simulink model "nav_filter"  (R2025b)
settings: Solver=ode4  StartTime=0.0  StopTime=50  FixedStep=ST  RelTol=1e-3
InitFcn:
  | addpath(genpath('KF_utilities'));
values from neighbouring files (symbols this model uses):
  acc = acc_f    [TRAJECTORY1.m]
  bias_gyro = [1 1 1]    [TRAJECTORY1.m]
  g = Simulink.Parameter    [TRAJECTORY1.m]
  P_bases_ned = Simulink.Parameter    [TRAJECTORY1.m]
  pos = pos_f    [TRAJECTORY1.m]
  pqr = omega_n    [TRAJECTORY1.m]
  Q = Simulink.Parameter    [TRAJECTORY1.m]
  quat_nb = compact(quat)    [TRAJECTORY1.m]
  sensor_covariances = Simulink.Parameter    [TRAJECTORY1.m]
  ST = 1/100    (= 0.01)    [TRAJECTORY1.m]    (also in WP_High_acc.m; WP_low_acc.m)
  vel_ned = vel_n_f    [TRAJECTORY1.m]
undefined symbols (not defined in the file or in its folder): DiscIntNeverNeededParam, freq_gyro, freq_UWB, N_bases, std_dev_gyro1, std_dev_gyro2, std_dev_gyro3, std_dev_magx, std_dev_magy, std_dev_magz, std_dev_UWB1, Tf
libraries: cstblocks x8, simulink x1
settings Model: Creator=eugde  LastModifiedBy=eugde

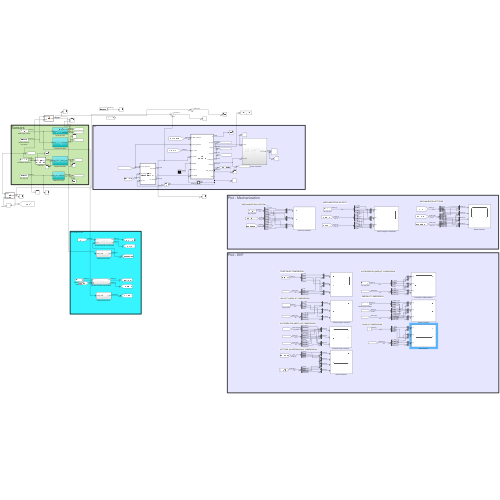
[thumbnail: Simulink's stored preview of the top-level diagram]
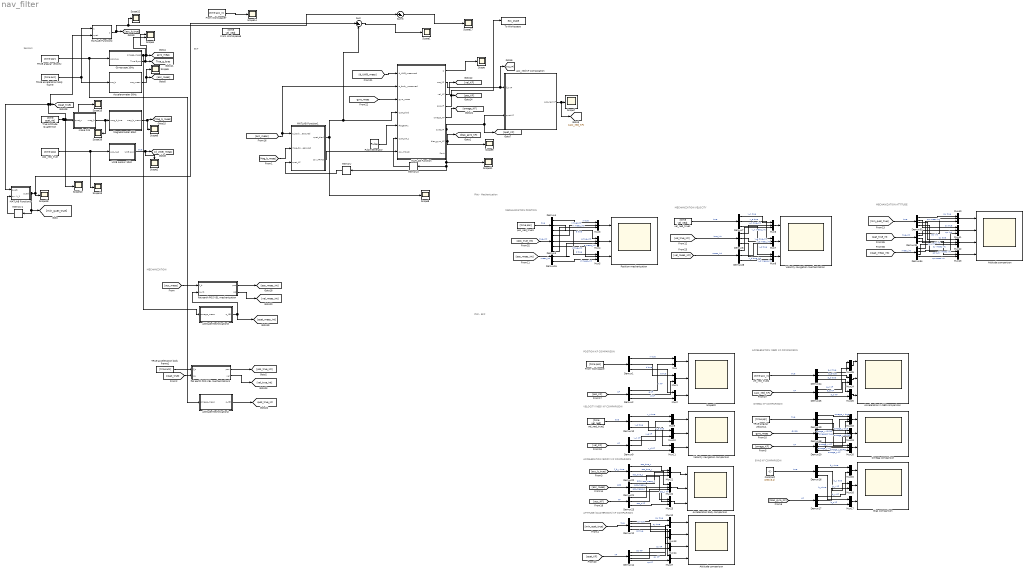
== system nav_filter ==
  note: MECHANIZATION
  note: EKF
  note: Sensors
  note: VELOCITY (NED) KF COMPARISON
  note: Plot - Mechanization
  note: MECHANIZATION VELOCITY
  note: OMEGA KF COMPARISON
  note: ACCELERATION (BODY) KF COMPARISON
  note: Plot - EKF
  note: POSITION KF COMPARISON
  note: MECHANIZATION POSITION
  note: BYAS KF COMPARISON
  note: ACCELERATION (NED) KF COMPARISON
  note: MECHANIZATION ATTITUDE
  note: ATTITUDE (QUATERNION) KF COMPARISON
  Acceleration body comparison : Scope  NumInputPorts=3
      settings: ActiveDisplayYMinimum=-4.52669  ActiveDisplayYMaximum=3.39128  YLabel=acc_x [m/s^2]
  Acceleration in NED comparison : Scope  NumInputPorts=3
      settings: ActiveDisplayYMinimum=-1.28826  ActiveDisplayYMaximum=1.68364  YLabel=acc_n [m/s^2]  DataLoggingVariableName=ScopeData2
  Accelerometer 50Hz : Subsystem
  Attitude Mechnization2 : Subsystem
  Attitude Mechnization3 : Subsystem
  "Attitude comparison " : Scope  NumInputPorts=4
      settings: ActiveDisplayYMinimum=-0.55605  ActiveDisplayYMaximum=1.17289  YLabel=qw  DataLoggingVariableName=ScopeData4
  "Attitude comparison " : Scope  NumInputPorts=4
      settings: ActiveDisplayYMinimum=-0.59703  ActiveDisplayYMaximum=1.17766  YLabel=qw  DataLoggingVariableName=ScopeData5
  Bias comparison : Scope  NumInputPorts=3
      settings: ActiveDisplayYMinimum=0.42457  ActiveDisplayYMaximum=1.1239  YLabel=bias_x [rad/s]  DataLoggingVariableName=ScopeData6
  Constant : Constant  Value=ones(3,1)
  Demux{1..4,6..7,9..10,15..25,28} (20 alike) : Demux  Outputs=3
  Demux{12,14,32..34} (5 alike) : Demux
  From Workspace : FromWorkspace  VariableName=[time pos]
  From Workspace6 : FromWorkspace  VariableName=[time vel_ned]
  From Workspace7 : FromWorkspace  VariableName=[time acc_n]
  Gyroscope 10Hz : Subsystem
  MATLAB Function : MATLAB Function  InitFcn=addpath('C:\Users\eugde\OneDrive\Documenti\Uni Pisa\Esami\SGN\PROGETTO\KF_utilities')  TreatAsAtomicUnit=on
  MATLAB Function1 : MATLAB Function  TreatAsAtomicUnit=on
  MATLAB Function2 : MATLAB Function  TreatAsAtomicUnit=on
  MATLAB Function3 : MATLAB Function  TreatAsAtomicUnit=on
  Magnetometer 50Hz : Subsystem
  Memory : Memory
  Memory1 : Memory  InitialCondition=quat_nb(1,:)
  Memory2 : Memory  InitialCondition=[1 0 0 0]'
  Mux{,1..2,9..17,24..27} (16 alike) : Mux  Inputs=2
  Mux{3..8,18..23,40..43} (16 alike) : Mux  Inputs=3
  Omega comparison : Scope  NumInputPorts=3
      settings: ActiveDisplayYMinimum=-0.27702  ActiveDisplayYMaximum=1.31187  YLabel=omega_x [rad/s]  DataLoggingVariableName=ScopeData7
  Position mechanization : Scope  NumInputPorts=3
      settings: ActiveDisplayYMinimum=-9.13016  ActiveDisplayYMaximum=45.84035  YLabel=North [m]  DataLoggingVariableName=ScopeData8
  Pulse Generator : DiscretePulseGenerator  PulseType=Time based  Period=1/50  PulseWidth=50
  Scope{,1..2,5..18} (17 alike) : Scope
      Scope settings: ActiveDisplayYMinimum=726.13831  ActiveDisplayYMaximum=1136.65509
      Scope1 settings: ActiveDisplayYMinimum=-0.05537  ActiveDisplayYMaximum=0.0472
      Scope10 settings: ActiveDisplayYMinimum=-1.54993  ActiveDisplayYMaximum=1.58064
      Scope11 settings: ActiveDisplayYMinimum=-0.44551  ActiveDisplayYMaximum=1.21227  DataLoggingVariableName=ScopeData12
      Scope12 settings: ActiveDisplayYMinimum=-0.13409  ActiveDisplayYMaximum=0.09726  DataLoggingVariableName=ScopeData13
      Scope13 settings: ActiveDisplayYMinimum=-15.92056  ActiveDisplayYMaximum=36.67619  DataLoggingVariableName=ScopeData14
      Scope14 settings: ActiveDisplayYMinimum=-4.68451  ActiveDisplayYMaximum=4.54841  DataLoggingVariableName=ScopeData2
      Scope15 settings: ActiveDisplayYMinimum=-0.55552  ActiveDisplayYMaximum=1.17284
      Scope16 settings: ActiveDisplayYMinimum=-0.9809  ActiveDisplayYMaximum=1.11497  DataLoggingVariableName=ScopeData2
      Scope17 settings: ActiveDisplayYMinimum=-9.00868  ActiveDisplayYMaximum=9.03518  DataLoggingVariableName=ScopeData2
      Scope18 settings: ActiveDisplayYMinimum=-0.55552  ActiveDisplayYMaximum=1.17284
      Scope2 settings: ActiveDisplayYMinimum=1.85826  ActiveDisplayYMaximum=83.14894  DataLoggingVariableName=ScopeData4
      Scope5 settings: ActiveDisplayYMinimum=-11.04684  ActiveDisplayYMaximum=1.25671  DataLoggingVariableName=ScopeData6
      Scope6 settings: ActiveDisplayYMinimum=-0.9809  ActiveDisplayYMaximum=1.11497  DataLoggingVariableName=ScopeData7
      Scope7 settings: ActiveDisplayYMinimum=-0.90235  ActiveDisplayYMaximum=0.76851  DataLoggingVariableName=ScopeData3
      Scope8 settings: ActiveDisplayYMinimum=-1.24871  ActiveDisplayYMaximum=1.24986
      Scope9 settings: ActiveDisplayYMinimum=0.05252  ActiveDisplayYMaximum=2.64364  DataLoggingVariableName=ScopeData5
  Scope20 : Scope  NumInputPorts=3
      settings: ActiveDisplayYMinimum=-3.73177  ActiveDisplayYMaximum=33.62683  YLabel=North  DataLoggingVariableName=ScopeData9
  Scope4 : Scope  NumInputPorts=2
      settings: ActiveDisplayYMinimum=0.99965  ActiveDisplayYMaximum=1.00021  DataLoggingVariableName=ScopeData5
  Sum : Sum  Inputs=|+-
  Sum3 : Sum  Inputs=|+-
  TRUE acceleration body frame : FromWorkspace  VariableName=[time acc]  SampleTime=ST
  TRUE acceleration body frame1 : FromWorkspace  VariableName=[time acc]  SampleTime=ST
  TRUE angular velocity : FromWorkspace  VariableName=[time pqr]  SampleTime=ST
  TRUE angular velocity1 : FromWorkspace  VariableName=[time pqr]  SampleTime=ST
  To Workspace : ToWorkspace  VariableName=ecs_state  SaveFormat=Structure With Time  SampleTime=-1
  True Attitude Quaternion : FromWorkspace  VariableName=[time quat_nb]  SampleTime=ST
  UWB sensor 10Hz : Subsystem
  Velocity navigation comparison : Scope  NumInputPorts=3
      settings: ActiveDisplayYMinimum=-0.23511  ActiveDisplayYMaximum=1.32366  YLabel=vel_n [m/s]  DataLoggingVariableName=ScopeData10
  Velocity navigation mechanization : Scope  NumInputPorts=3
      settings: ActiveDisplayYMinimum=0.32185  ActiveDisplayYMaximum=0.95452  YLabel=vel_n [m/s]  DataLoggingVariableName=ScopeData11
  "acc_ned KF computation " : Subsystem
  flat earth POS VEL mechanization : Subsystem
  flat earth POS VEL mechanization1 : Subsystem
  make Cnb : MATLAB Function  TreatAsAtomicUnit=on
  pos_ned_true : FromWorkspace  VariableName=[time pos]  SampleTime=ST
  pos_ned_true1 : FromWorkspace  VariableName=[time pos]  SampleTime=ST
  vel_ned_true1 : FromWorkspace  VariableName=[time vel_ned]  SampleTime=ST
  vel_ned_true2 : FromWorkspace  VariableName=[time vel_ned]  SampleTime=ST
  vel_ned_true4 : FromWorkspace  VariableName=[time acc_n]  SampleTime=ST
  tag scope: True_g_byas=global, gyro_meas=global, quat_true_int=global
  wires:
  Magnetometer 50Hz/1(mag_b_meas) -> Scope6/1, [Mag_b_meas]
  True Attitude Quaternion/1 -> Scope10/1, MATLAB Function3/1("quatk "), MATLAB Function2/2(quat), [quat_true], Scope15/1, make Cnb/1(quat_n)
  Gyroscope 10Hz/2(True Byas) -> Scope4/2, [True_g_byas]
  Gyroscope 10Hz/1(omega_meas) -> Attitude Mechnization3/1(omega_meas), [gyro_meas], Scope4/1
  pos_ned_true/1 -> Scope13/1, UWB sensor 10Hz/1(pos_ned)
  Accelerometer 50Hz/1(acc_meas) -> Scope5/1, [acc_meas]
  TRUE angular velocity/1 -> Attitude Mechnization2/1(omega_meas), Gyroscope 10Hz/1(pqr_true)
  TRUE acceleration body frame/1 -> MATLAB Function2/1(acc_meas), Accelerometer 50Hz/1(acc_b)
  UWB sensor 10Hz/1("UWB pos ") -> Scope2/1, [d_UWB_meas]  "true"
  "acc_ned KF computation "/1(acc_ned KF) -> [acc_ned_KF], Scope7/1
  MATLAB Function/6(quat_KF) -> Scope11/1, Memory2/1, Memory/1, [quat_KF], "acc_ned KF computation "/2(quat KF)
  [acc_meas] -> MATLAB Function/2(a_body_measured), MATLAB Function1/1(a_body_measured)
  MATLAB Function/7(bias_gyro_KF) -> [bias_gyro_KF], Scope9/1
  MATLAB Function/5(omega_KF) -> [omega_KF]
  MATLAB Function/4(pos_KF) -> To Workspace/1, [pos_KF]
  [gyro_meas] -> MATLAB Function/3(gyro_meas)
  [d_UWB_meas] -> MATLAB Function/1(d_UWB_measured)
  make Cnb/1(mag_b) -> Scope16/1, Magnetometer 50Hz/1(mag_b_true)
  MATLAB Function1/1(quat_triad) -> Scope8/1, Sum/2, MATLAB Function/4(quat_triad)
  [Mag_b_meas] -> MATLAB Function1/2(mag_body_measured)
  MATLAB Function/3(vel_KF) -> [vel_KF]
  MATLAB Function/2(acc_KF) -> [acc_KF], "acc_ned KF computation "/1(f_b KF)
  [acc_meas] -> flat earth POS VEL mechanization/1(f_b)
  Attitude Mechnization3/1(q_NB) -> [quat_meas_int], flat earth POS VEL mechanization/2(q_nb)
  Memory/1 -> MATLAB Function1/3(quat_KF)
  From Workspace7/1 -> Scope14/1
  Sum3/1 -> Scope17/1
  Sum/1 -> Scope1/1
  MATLAB Function3/1(quatk) -> [min_quat_true], Memory1/1, Sum/1, Scope18/1
  Memory1/1 -> MATLAB Function3/2(quatk_1)
  Memory2/1 -> MATLAB Function/6(quat_KF_1)
  MATLAB Function/1(Z) -> Scope/1
  Mux8/1 -> Velocity navigation mechanization/3
  [bias_gyro_KF] -> Demux17/1  "KF"
  Demux14/1 -> Mux12/2  "qw KF"
  Demux19/2 -> Mux19/1  "omega_y true"
  Demux23/2 -> Mux22/3  "acc_y KF"
  Mux16/1 -> Bias comparison/2
  Demux17/2 -> Mux16/2  "b_y KF"
  [pos_true_int] -> Demux3/1  "true_int"
  Demux1/3 -> Mux2/1  "d true"
  Demux14/3 -> Mux14/2  "qy KF"
  Demux33/4 -> Mux43/1  "qz true"
  [vel_true_int] -> Demux6/1  "true_int"
  [quat_KF] -> Demux14/1  "KF"
  Mux9/1 -> Velocity navigation comparison/1
  Mux24/1 -> Acceleration in NED comparison/2
  Mux19/1 -> Omega comparison/2
  [pos_KF] -> Demux2/1  "KF"
  Demux7/3 -> Mux8/1  "v_d true"
  Demux6/3 -> Mux8/2  "v_d true_int"
  Demux7/2 -> Mux7/1  "v_e true"
  Demux20/3 -> Mux20/3  "omega_z KF"
  Mux15/1 -> Bias comparison/1
  Demux16/2 -> Mux16/1  "b_y true"
  Demux1/1 -> Mux/1  "n true"
  Demux24/3 -> Mux25/1  "a_d true"
  Demux9/3 -> Mux11/2  "v_d KF"
  Constant/1 -> Demux16/1  "true"
  Mux11/1 -> Velocity navigation comparison/3
  [min_quat_true] -> Demux12/1  "true"
  Mux1/1 -> Scope20/2
  From Workspace/1 -> Demux1/1
  Mux22/1 -> Acceleration body comparison/2
  Mux5/1 -> Position mechanization/3
  Mux41/1 -> "Attitude comparison "/2
  Demux33/1 -> Mux40/1  "qw true"
  Mux/1 -> Scope20/1
  Demux4/3 -> Mux5/1  "d true"
  Mux6/1 -> Velocity navigation mechanization/1
  Mux27/1 -> "Attitude comparison "/4
  Mux14/1 -> "Attitude comparison "/3
  Demux20/1 -> Mux18/3  "omega_x KF"
  Mux18/1 -> Omega comparison/1
  Demux22/2 -> Mux22/1  "acc_true_y"
  Demux17/3 -> Mux17/2  "b_z KF"
  TRUE angular velocity1/1 -> Demux19/1  "true"
  Demux21/2 -> Mux22/2  "acc_meas_y"
  Demux7/1 -> Mux6/1  "v_n true"
  vel_ned_true1/1 -> Demux7/1  "true"
  Demux16/3 -> Mux17/1  "b_z true"
  Mux25/1 -> Acceleration in NED comparison/3
  [vel_KF] -> Demux9/1  "KF"
  Demux17/1 -> Mux15/2  "b_x KF"
  Demux9/1 -> Mux9/2  "v_n KF"
  Demux3/2 -> Mux4/2  "e true_int"
  Mux2/1 -> Scope20/3
  Demux3/3 -> Mux5/2  "d true_int"
  Demux3/1 -> Mux3/2  "n true_int"
  Demux24/2 -> Mux24/1  "a_e true"
  Demux6/2 -> Mux7/2  "v_e true_int"
  Mux26/1 -> Acceleration in NED comparison/1
  Demux33/3 -> Mux42/1  "qy true"
  [acc_meas] -> Demux21/1  "ACC"
  Demux32/1 -> Mux40/2  "qw int"
  Demux25/1 -> Mux26/2  "a_n KF"
  Demux19/1 -> Mux18/1  "omega_x true"
  Demux16/1 -> Mux15/1  "b_x true"
  Demux21/3 -> Mux23/2  "acc_meas_z"
  Demux10/3 -> Mux11/1  "v_d true"
  Mux17/1 -> Bias comparison/3
  Demux25/2 -> Mux24/2  "a_e KF"
  Mux20/1 -> Omega comparison/3
  Demux12/2 -> Mux13/1  "qx true"
  Demux32/4 -> Mux43/2  "qz int"
  pos_ned_true1/1 -> Demux4/1  "true"
  Demux32/2 -> Mux41/2  "qw int"
  Mux23/1 -> Acceleration body comparison/3
  vel_ned_true4/1 -> Demux24/1  "true"
  Demux14/2 -> Mux13/2  "qx KF"
  [min_quat_true] -> Demux33/1  "true"
  vel_ned_true2/1 -> Demux10/1  "true"
  Demux10/1 -> Mux9/1  "v_n true"
  Demux4/2 -> Mux4/1  "e true"
  Mux12/1 -> "Attitude comparison "/1
  Mux10/1 -> Velocity navigation comparison/2
  Mux43/1 -> "Attitude comparison "/4
  Demux33/2 -> Mux41/1  "qx true"
  Demux23/1 -> Mux21/3  "acc_x KF"
  Demux19/3 -> Mux20/1  "omega_z true"
  Demux23/3 -> Mux23/3  "acc_z KF"
  Demux6/1 -> Mux6/2  "v_n true_int"
  Demux2/3 -> Mux2/2  "d KF"
  Demux10/2 -> Mux10/1  "v_e true"
  Demux1/2 -> Mux1/1  "e true"
  Demux24/1 -> Mux26/1  "a_n true"
  Mux4/1 -> Position mechanization/2
  Demux20/2 -> Mux19/3  "omega_y KF"
  Demux32/3 -> Mux42/2  "qy int"
  Demux9/2 -> Mux10/2  "v_e KF"
  [acc_b_true] -> Demux22/1  "f_b_y true"
  [acc_ned_KF] -> Demux25/1  "KF"
  [omega_KF] -> Demux20/1  "KF"
  Demux4/1 -> Mux3/1  "n true"
  Mux42/1 -> "Attitude comparison "/3
  Mux13/1 -> "Attitude comparison "/2
  Mux21/1 -> Acceleration body comparison/1
  [acc_KF] -> Demux23/1  "KF"
  Demux2/2 -> Mux1/2  "e KF"
  [quat_true_int] -> Demux32/1  "true_int"
  Demux14/4 -> Mux27/2  "qz KF"
  Demux22/3 -> Mux23/1  "acc_true_z"
  Demux12/1 -> Mux12/1  "qw true"
  Demux25/3 -> Mux25/2  "a_d KF"
  Mux40/1 -> "Attitude comparison "/1
  Demux22/1 -> Mux21/1  "acc_true_x"
  Demux12/3 -> Mux14/1  "qy true"
  Demux21/1 -> Mux21/2  "acc_meas_x"
  Mux3/1 -> Position mechanization/1
  Demux2/1 -> Mux/2  "n KF"
  Mux7/1 -> Velocity navigation mechanization/2
  flat earth POS VEL mechanization/1(pos) -> [pos_meas_int]
  flat earth POS VEL mechanization/2(vel) -> [vel_meas_int]
  Attitude Mechnization2/1(q_NB) -> [quat_true_int]
  MATLAB Function2/1(acc_body) -> [acc_b_true], Scope12/1, Sum3/1
  flat earth POS VEL mechanization1/1(pos) -> [pos_true_int]
  flat earth POS VEL mechanization1/2(vel) -> [vel_true_int]
  [quat_true] -> flat earth POS VEL mechanization1/2(rpy)
  Demux12/4 -> Mux27/1  "qz true"
  TRUE acceleration body frame1/1 -> flat earth POS VEL mechanization1/1(f_b)
  [gyro_meas] -> Demux18/1  "GYRO"
  Demux18/1 -> Mux18/2  "omega_x GYRO"
  Demux18/2 -> Mux19/2  "omega_y GYRO"
  Demux18/3 -> Mux20/2  "omega_z GYRO"
  MATLAB Function1/2(cov_TRIAD) -> MATLAB Function/7(cov_TRIAD)
  Pulse Generator/1 -> MATLAB Function/5(Flag50Hz)
  [pos_meas_int] -> Demux15/1  "meas_int"
  Demux28/2 -> Mux7/3  "v_e meas_int"
  Demux28/3 -> Mux8/3  "v_d meas_int"
  Demux34/3 -> Mux42/3  "qy meas int"
  Demux15/2 -> Mux4/3  "e meas_int"
  Demux34/4 -> Mux43/3  "qz meas int"
  Demux15/3 -> Mux5/3  "d meas_int"
  [vel_meas_int] -> Demux28/1  "meas_int"
  Demux15/1 -> Mux3/3  "n meas_int"
  Demux28/1 -> Mux6/3  "v_n meas_int"
  [quat_meas_int] -> Demux34/1  "meas_int"
  Demux34/1 -> Mux40/3  "qw meas int"
  Demux34/2 -> Mux41/3  "qx meas int"

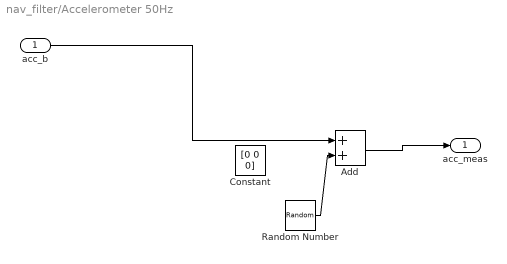
== system nav_filter/Accelerometer 50Hz ==
  acc_b : Inport
  Add : Sum
  Constant : Constant  Value=[0 0 0]
  Random Number : RandomNumber  Mean=zeros(1,3)  Variance=sensor_covariances(end-9:end-7)  SampleTime=0.1
  acc_meas : Outport
  wires:
  Add/1 -> acc_meas/1
  acc_b/1 -> Add/1
  Random Number/1 -> Add/2

== system nav_filter/Attitude Mechnization2 ==
  omega_meas : Inport
  Delay : Delay  DelayLength=1  InitialCondition=quat_nb(1,:)
  quaternion update : MATLAB Function  TreatAsAtomicUnit=on
  q_NB : Outport
  wires:
  omega_meas/1 -> quaternion update/1(omega_meas)
  quaternion update/1(new_quat) -> q_NB/1, Delay/1
  Delay/1 -> quaternion update/2(q_NB)

== system nav_filter/Attitude Mechnization3 ==
  omega_meas : Inport
  Delay : Delay  DelayLength=1  InitialCondition=quat_nb(1,:)
  quaternion update : MATLAB Function  TreatAsAtomicUnit=on
  q_NB : Outport
  wires:
  omega_meas/1 -> quaternion update/1(omega_meas)
  quaternion update/1(new_quat) -> q_NB/1, Delay/1
  Delay/1 -> quaternion update/2(q_NB)

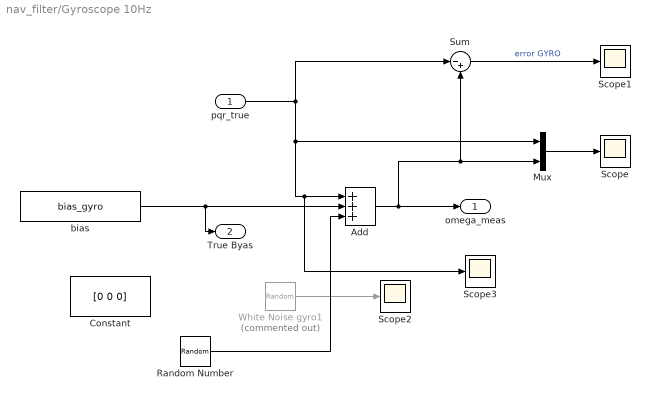
== system nav_filter/Gyroscope 10Hz ==
  pqr_true : Inport
  Add : Sum  Inputs=+++
  Constant : Constant  Value=[0 0 0]
  Mux : Mux  Inputs=2
  Random Number : RandomNumber  Mean=zeros(1,3)  Variance=sensor_covariances(end-2:end)'  SampleTime=0.01
  Scope{,1..3} (4 alike) : Scope
      Scope settings: ActiveDisplayYMinimum=-0.1418  ActiveDisplayYMaximum=0.20182  YLabel=[rad/s]  DataLoggingVariableName=ScopeData2
      Scope1 settings: ActiveDisplayYMinimum=0.9  ActiveDisplayYMaximum=1.1  DataLoggingVariableName=ScopeData23
      Scope2 settings: ActiveDisplayYMinimum=-0.0134  ActiveDisplayYMaximum=0.01406  DataLoggingVariableName=ScopeData6
      Scope3 settings: ActiveDisplayYMinimum=-0.00035  ActiveDisplayYMaximum=0.00021  DataLoggingVariableName=ScopeData2
  Sum : Sum  Inputs=|-+
  White Noise gyro1 : RandomNumber  Commented=on  DisableCoverage=on  Mean=[0 0 0]  Variance=[std_dev_gyro1,std_dev_gyro2,std_dev_gyro3]  Seed=[4 5 6]  SampleTime=1/freq_gyro
  bias : Constant  Value=bias_gyro  SampleTime=ST
  omega_meas : Outport
  True Byas : Outport  Port=2
  wires:
  Mux/1 -> Scope/1
  pqr_true/1 -> Mux/1, Scope3/1, Add/1, Sum/1
  White Noise gyro1/1 -> Scope2/1
  Add/1 -> Sum/2, Mux/2, omega_meas/1
  Sum/1 -> Scope1/1  "error GYRO"
  bias/1 -> True Byas/1, Add/2
  Random Number/1 -> Add/3

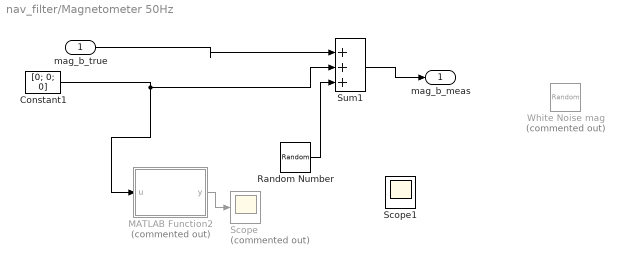
== system nav_filter/Magnetometer 50Hz ==
  mag_b_true : Inport
  Constant1 : Constant  Value=[0; 0; 0]
  MATLAB Function2 : MATLAB Function  Commented=on  TreatAsAtomicUnit=on
  Random Number : RandomNumber  Mean=[0;0;0]  Variance=[1e-4;1e-4;1e-4]  SampleTime=0.01
  Scope : Scope  Commented=on
  Scope1 : Scope
      settings: ActiveDisplayYMinimum=-0.15329  ActiveDisplayYMaximum=0.15128  DataLoggingVariableName=ScopeData2
  Sum1 : Sum  Inputs=|+++
  White Noise mag : RandomNumber  Commented=on  DisableCoverage=on  Mean=[0 0 0]  Variance=[std_dev_magx^2, std_dev_magy^2, std_dev_magz^2]  Seed=[7 8 9]  SampleTime=Tf
  mag_b_meas : Outport
  wires:
  mag_b_true/1 -> Sum1/1
  ? -> ?
  Constant1/1 -> MATLAB Function2/1(u), Sum1/2
  Sum1/1 -> mag_b_meas/1
  MATLAB Function2/1(y) -> Scope/1
  Random Number/1 -> Sum1/3

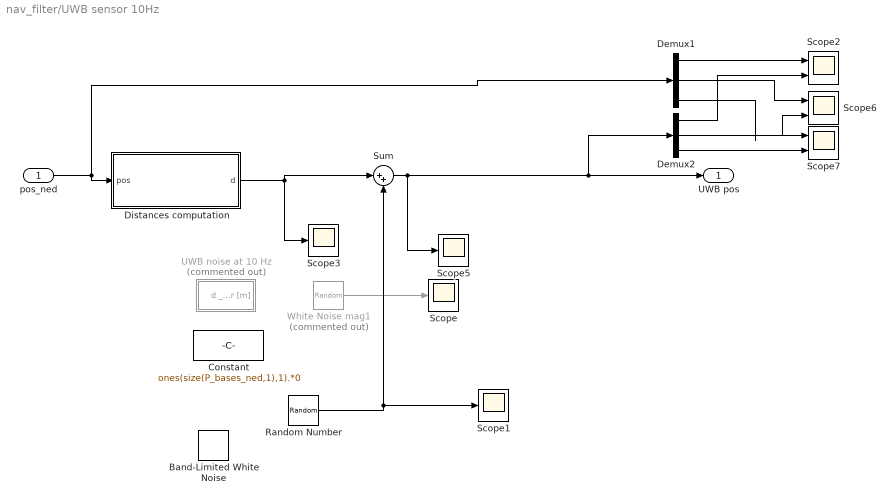
== system nav_filter/UWB sensor 10Hz ==
  pos_ned : Inport  PortDimensions=3
  Band-Limited White Noise : simulink/Sources/Band-Limited White Noise  Cov=sensor_covariances(1:size(P_bases_ned,1))'  Ts=0.01  seed=[23341]
  Constant : Constant  Value=ones(size(P_bases_ned,1),1).*0
  Demux1 : Demux  Outputs=3
  Demux2 : Demux  Outputs=3
  Distances computation : MATLAB Function  TreatAsAtomicUnit=on
  Random Number : RandomNumber  Mean=zeros(1,size(P_bases_ned,1))  Variance=sensor_covariances(1:size(P_bases_ned,1))'  SampleTime=0.01
  Scope{,1,3,5} (4 alike) : Scope
      Scope settings: ActiveDisplayYMinimum=-0.38772  ActiveDisplayYMaximum=0.448
      Scope1 settings: ActiveDisplayYMinimum=-0.09862  ActiveDisplayYMaximum=0.09586  DataLoggingVariableName=ScopeData3
      Scope3 settings: ActiveDisplayYMinimum=-946.03158  ActiveDisplayYMaximum=8514.28426  DataLoggingVariableName=ScopeData14
      Scope5 settings: ActiveDisplayYMinimum=1001.9626  ActiveDisplayYMaximum=1002.6  DataLoggingVariableName=ScopeData8
  Scope2 : Scope  NumInputPorts=2
      settings: ActiveDisplayYMinimum=14.63738  ActiveDisplayYMaximum=68.36896  DataLoggingVariableName=ScopeData4
  Scope6 : Scope  NumInputPorts=2
      settings: ActiveDisplayYMinimum=-364.79349  ActiveDisplayYMaximum=3275.37823  DataLoggingVariableName=ScopeData3
  Scope7 : Scope  NumInputPorts=2
      settings: ActiveDisplayYMinimum=-9.37061  ActiveDisplayYMaximum=84.33547  DataLoggingVariableName=ScopeData5
  Sum : Sum  Inputs=|++
  UWB noise at 10 Hz : Subsystem  Commented=on  mask{AMPd1=5, AMPd2=5, AMPd3=5, AMPd4=5, newnoise=on, seed_user=0}
      mask prompts: AMPd1 "UWB approx max error d1 [m]"; AMPd2 "UWB approx max error d2 [m]"; AMPd3 "UWB approx max error d3 [m]"; AMPd4 "UWB approx max error d4 [m]"; newnoise "new noise at each run"; seed_user "user provided seed value"
      mask init:
      | if newnoise,
      |         seedx=rand(1)*1000;
      |         seedy=rand(1)*1000;
      |         seedz=rand(1)*1000;
      |     else
      |         seedx=seed_user;
      |         seedy=seed_user+1;
      |         seedz=seed_user+2;
      |     end
      mask DialogControl ParameterGroupVar Prompt: Noise generation
  White Noise mag1 : RandomNumber  Commented=on  DisableCoverage=on  Mean=zeros(N_bases,1)  Variance=std_dev_UWB1*ones(N_bases,1)  Seed=7:7+N_bases-1  SampleTime=1/freq_UWB
  "UWB pos " : Outport
  wires:
  pos_ned/1 -> Demux1/1, Distances computation/1(pos)
  White Noise mag1/1 -> Scope/1
  Demux2/2 -> Scope6/2
  Demux1/2 -> Scope6/1
  Demux1/1 -> Scope2/1
  Demux2/1 -> Scope2/2
  Demux1/3 -> Scope7/1
  Demux2/3 -> Scope7/2
  Sum/1 -> "UWB pos "/1, Demux2/1, Scope5/1
  Distances computation/1(d) -> Sum/1, Scope3/1
  Random Number/1 -> Sum/2, Scope1/1

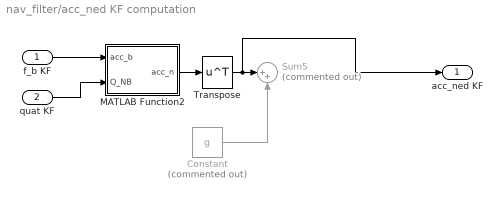
== system nav_filter/acc_ned KF computation  ==
  f_b KF : Inport
  quat KF : Inport  Port=2
  Constant : Constant  Commented=on  Value=g
  MATLAB Function2 : MATLAB Function  TreatAsAtomicUnit=on
  Sum5 : Sum  Commented=on  Inputs=|++
  Transpose : Math  Operator=transpose
  acc_ned KF : Outport
  wires:
  quat KF/1 -> MATLAB Function2/2(Q_NB)
  f_b KF/1 -> MATLAB Function2/1(acc_b)
  Constant/1 -> Sum5/2
  MATLAB Function2/1(acc_n) -> Transpose/1
  Transpose/1 -> acc_ned KF/1, Sum5/1

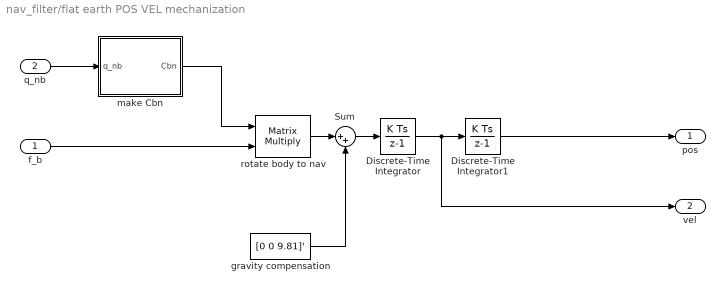
== system nav_filter/flat earth POS VEL mechanization ==
  f_b : Inport
  q_nb : Inport  Port=2
  Discrete-Time Integrator : DiscreteIntegrator  InitialCondition=vel_ned(1,:)  SampleTime=-1  ICPrevOutput=DiscIntNeverNeededParam  ICPrevScaledInput=DiscIntNeverNeededParam
  Discrete-Time Integrator1 : DiscreteIntegrator  InitialCondition=pos(1,:)  SampleTime=-1  ICPrevOutput=DiscIntNeverNeededParam  ICPrevScaledInput=DiscIntNeverNeededParam
  Sum : Sum  Inputs=|++
  gravity compensation : Constant  Value=[0 0 9.81]'
  make Cbn : MATLAB Function  TreatAsAtomicUnit=on
  rotate body to nav : Product  Multiplication=Matrix(*)
  pos : Outport
  vel : Outport  Port=2
  wires:
  rotate body to nav/1 -> Sum/1
  gravity compensation/1 -> Sum/2
  Discrete-Time Integrator/1 -> vel/1, Discrete-Time Integrator1/1
  make Cbn/1(Cbn) -> rotate body to nav/1
  Discrete-Time Integrator1/1 -> pos/1
  Sum/1 -> Discrete-Time Integrator/1
  f_b/1 -> rotate body to nav/2
  q_nb/1 -> make Cbn/1(q_nb)

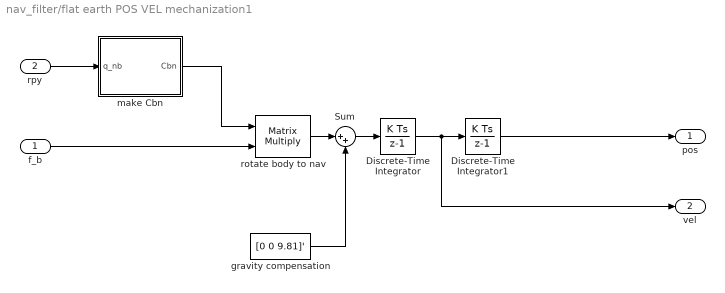
== system nav_filter/flat earth POS VEL mechanization1 ==
  f_b : Inport
  rpy : Inport  Port=2
  Discrete-Time Integrator : DiscreteIntegrator  InitialCondition=vel_ned(1,:)'  SampleTime=-1  ICPrevOutput=DiscIntNeverNeededParam  ICPrevScaledInput=DiscIntNeverNeededParam
  Discrete-Time Integrator1 : DiscreteIntegrator  InitialCondition=pos(1,:)'  SampleTime=-1  ICPrevOutput=DiscIntNeverNeededParam  ICPrevScaledInput=DiscIntNeverNeededParam
  Sum : Sum  Inputs=|++
  gravity compensation : Constant  Value=[0 0 9.81]'
  make Cbn : MATLAB Function  TreatAsAtomicUnit=on
  rotate body to nav : Product  Multiplication=Matrix(*)
  pos : Outport
  vel : Outport  Port=2
  wires:
  rotate body to nav/1 -> Sum/1
  gravity compensation/1 -> Sum/2
  Discrete-Time Integrator/1 -> vel/1, Discrete-Time Integrator1/1
  make Cbn/1(Cbn) -> rotate body to nav/1
  Discrete-Time Integrator1/1 -> pos/1
  Sum/1 -> Discrete-Time Integrator/1
  f_b/1 -> rotate body to nav/2
  rpy/1 -> make Cbn/1(q_nb)

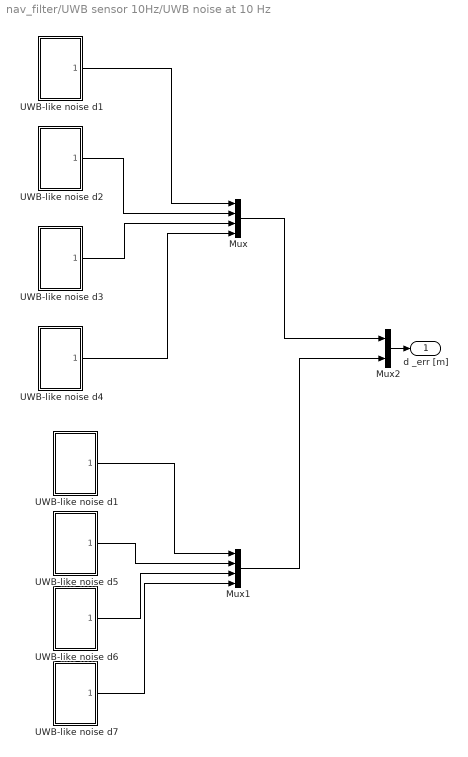
== system nav_filter/UWB sensor 10Hz/UWB noise at 10 Hz ==
  Mux : Mux
  Mux1 : Mux
  Mux2 : Mux  Inputs=2
  UWB-like noise d1 : Subsystem
  "UWB-like noise d1 " : Subsystem
  UWB-like noise d2 : Subsystem
  UWB-like noise d3 : Subsystem
  UWB-like noise d4 : Subsystem
  UWB-like noise d5 : Subsystem
  UWB-like noise d6 : Subsystem
  UWB-like noise d7 : Subsystem
  d _err [m] : Outport
  wires:
  "UWB-like noise d1 "/1(d1_err) -> Mux/1
  Mux/1 -> Mux2/1
  UWB-like noise d2/1(d2_err) -> Mux/2
  UWB-like noise d3/1(d3_err) -> Mux/3
  UWB-like noise d4/1(d4_err) -> Mux/4
  Mux1/1 -> Mux2/2
  UWB-like noise d1/1(d4_err) -> Mux1/1
  UWB-like noise d5/1(d4_err) -> Mux1/2
  UWB-like noise d6/1(d4_err) -> Mux1/3
  UWB-like noise d7/1(d4_err) -> Mux1/4
  Mux2/1 -> d _err [m]/1

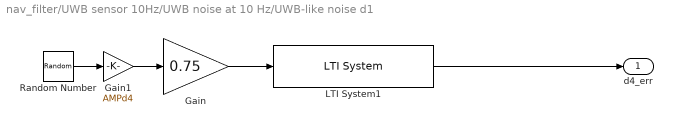
== system nav_filter/UWB sensor 10Hz/UWB noise at 10 Hz/UWB-like noise d1 ==
  Gain : Gain  Gain=0.75
  Gain1 : Gain  Gain=AMPd4
  LTI System1 : cstblocks/LTI System  sys=c2d(tf(1,[0.75 1])*tf([3000 0],[3000 1]),1/10)  IC=[]  PadeOrder=0
  Random Number : RandomNumber  Variance=0.01  Seed=13  SampleTime=1/freq_UWB
  d4_err : Outport
  wires:
  Gain1/1 -> Gain/1
  Gain/1 -> LTI System1/1
  Random Number/1 -> Gain1/1
  LTI System1/1 -> d4_err/1

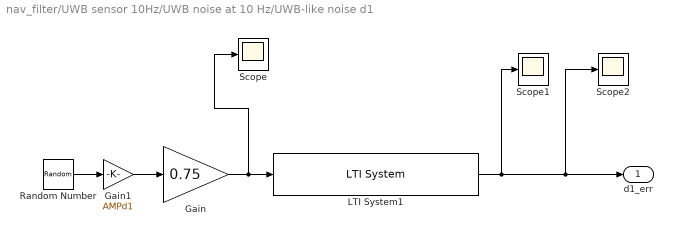
== system nav_filter/UWB sensor 10Hz/UWB noise at 10 Hz/UWB-like noise d1  ==
  Gain : Gain  Gain=0.75
  Gain1 : Gain  Gain=AMPd1
  LTI System1 : cstblocks/LTI System  sys=c2d(tf(1,[0.75 1])*tf([3000 0],[3000 1]),1/10)  IC=[]  PadeOrder=0
  Random Number : RandomNumber  Variance=0.01  Seed=10  SampleTime=1/freq_UWB
  Scope : Scope
      settings: ActiveDisplayYMinimum=-1.52728  ActiveDisplayYMaximum=1.65685  DataLoggingVariableName=ScopeData19
  Scope1 : Scope
      settings: ActiveDisplayYMinimum=-0.37838  ActiveDisplayYMaximum=0.40885  DataLoggingVariableName=ScopeData20
  Scope2 : Scope
      settings: ActiveDisplayYMinimum=-0.37838  ActiveDisplayYMaximum=0.40885  DataLoggingVariableName=ScopeData21
  d1_err : Outport
  wires:
  Gain1/1 -> Gain/1
  Gain/1 -> Scope/1, LTI System1/1
  Random Number/1 -> Gain1/1
  LTI System1/1 -> Scope2/1, d1_err/1, Scope1/1

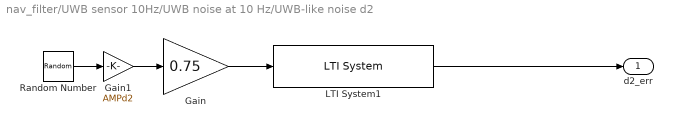
== system nav_filter/UWB sensor 10Hz/UWB noise at 10 Hz/UWB-like noise d2 ==
  Gain : Gain  Gain=0.75
  Gain1 : Gain  Gain=AMPd2
  LTI System1 : cstblocks/LTI System  sys=c2d(tf(1,[0.75 1])*tf([3000 0],[3000 1]),1/10)  IC=[]  PadeOrder=0
  Random Number : RandomNumber  Variance=0.01  Seed=11  SampleTime=1/freq_UWB
  d2_err : Outport
  wires:
  Gain1/1 -> Gain/1
  Gain/1 -> LTI System1/1
  Random Number/1 -> Gain1/1
  LTI System1/1 -> d2_err/1

== system nav_filter/UWB sensor 10Hz/UWB noise at 10 Hz/UWB-like noise d3 ==
  Gain : Gain  Gain=0.75
  Gain1 : Gain  Gain=AMPd3
  LTI System1 : cstblocks/LTI System  sys=c2d(tf(1,[0.75 1])*tf([3000 0],[3000 1]),1/10)  IC=[]  PadeOrder=0
  Random Number : RandomNumber  Variance=0.01  Seed=12  SampleTime=1/freq_UWB
  d3_err : Outport
  wires:
  Gain1/1 -> Gain/1
  Gain/1 -> LTI System1/1
  Random Number/1 -> Gain1/1
  LTI System1/1 -> d3_err/1

== system nav_filter/UWB sensor 10Hz/UWB noise at 10 Hz/UWB-like noise d4 ==
  Gain : Gain  Gain=0.75
  Gain1 : Gain  Gain=AMPd4
  LTI System1 : cstblocks/LTI System  sys=c2d(tf(1,[0.75 1])*tf([3000 0],[3000 1]),1/10)  IC=[]  PadeOrder=0
  Random Number : RandomNumber  Variance=0.01  Seed=13  SampleTime=1/freq_UWB
  d4_err : Outport
  wires:
  Gain1/1 -> Gain/1
  Gain/1 -> LTI System1/1
  Random Number/1 -> Gain1/1
  LTI System1/1 -> d4_err/1

== system nav_filter/UWB sensor 10Hz/UWB noise at 10 Hz/UWB-like noise d5 ==
  Gain : Gain  Gain=0.75
  Gain1 : Gain  Gain=AMPd4
  LTI System1 : cstblocks/LTI System  sys=c2d(tf(1,[0.75 1])*tf([3000 0],[3000 1]),1/10)  IC=[]  PadeOrder=0
  Random Number : RandomNumber  Variance=0.01  Seed=13  SampleTime=1/freq_UWB
  d4_err : Outport
  wires:
  Gain1/1 -> Gain/1
  Gain/1 -> LTI System1/1
  Random Number/1 -> Gain1/1
  LTI System1/1 -> d4_err/1

== system nav_filter/UWB sensor 10Hz/UWB noise at 10 Hz/UWB-like noise d6 ==
  Gain : Gain  Gain=0.75
  Gain1 : Gain  Gain=AMPd4
  LTI System1 : cstblocks/LTI System  sys=c2d(tf(1,[0.75 1])*tf([3000 0],[3000 1]),1/10)  IC=[]  PadeOrder=0
  Random Number : RandomNumber  Variance=0.01  Seed=13  SampleTime=1/freq_UWB
  d4_err : Outport
  wires:
  Gain1/1 -> Gain/1
  Gain/1 -> LTI System1/1
  Random Number/1 -> Gain1/1
  LTI System1/1 -> d4_err/1

== system nav_filter/UWB sensor 10Hz/UWB noise at 10 Hz/UWB-like noise d7 ==
  Gain : Gain  Gain=0.75
  Gain1 : Gain  Gain=AMPd4
  LTI System1 : cstblocks/LTI System  sys=c2d(tf(1,[0.75 1])*tf([3000 0],[3000 1]),1/10)  IC=[]  PadeOrder=0
  Random Number : RandomNumber  Variance=0.01  Seed=13  SampleTime=1/freq_UWB
  d4_err : Outport
  wires:
  Gain1/1 -> Gain/1
  Gain/1 -> LTI System1/1
  Random Number/1 -> Gain1/1
  LTI System1/1 -> d4_err/1

== matlab function nav_filter/make Cnb ==
  data: quat_n input; mag_b output; mag_n parameter
function mag_b = sim_mag_body(quat_n, mag_n)
quat_n = quat_n';

%define magnetic field and rotate to bodyframe
quat_n = quaternion(quat_n);
mag_b = rotmat(quat_n,"frame")* mag_n';

== matlab function nav_filter/flat earth POS VEL mechanization/make Cbn ==
  data: q_nb input; Cbn output
function Cbn = make_Cbn(q_nb)
%compute Cbn
q_nb  = quaternion(q_nb);
Cbn = quat2rotm(q_nb);

== matlab function nav_filter/Attitude Mechnization3/quaternion update ==
  data: omega_meas input; q_NB input; new_quat output; ST parameter
function new_quat = fcn(omega_meas, q_NB, ST)

omega_norm = norm(omega_meas);

if omega_norm < 1e-4  % or a small threshold
    delta_q = [1, 0, 0, 0];  % no rotation
else
    theta = double(omega_norm * ST);
    axis = double(omega_meas / omega_norm);
    delta_q = [cos(theta/2), axis' .* sin(theta/2)];
end

new_quat = quat_prod(q_NB,delta_q);
new_quat = new_quat / norm(new_quat);
end



function q = quat_prod(q1, q2)
    % q1, q2 are 1x4 vectors: [w x y z]
    w1 = q1(1); x1 = q1(2); y1 = q1(3); z1 = q1(4);
    w2 = q2(1); x2 = q2(2); y2 = q2(3); z2 = q2(4);

    w = w1*w2 - x1*x2 - y1*y2 - z1*z2;
    x = w1*x2 + x1*w2 + y1*z2 - z1*y2;
    y = w1*y2 - x1*z2 + y1*w2 + z1*x2;
    z = w1*z2 + x1*y2 - y1*x2 + z1*w2;

    q = [w, x, y, z];
end

== matlab function nav_filter/flat earth POS VEL mechanization1/make Cbn ==
  data: q_nb input; Cbn output
function Cbn = make_Cbn(q_nb)
%compute Cbn
q_nb  = quaternion(q_nb');
Cbn = quat2rotm((q_nb));

== matlab function nav_filter/acc_ned KF computation /MATLAB Function2 ==
  data: acc_b input; acc_n output; Q_NB input
function acc_n = fcn(acc_b,Q_NB)
Q_NB = conj(quaternion(Q_NB'));
acc_n = (rotmat(Q_NB,"frame")*acc_b)';

== matlab function nav_filter/Attitude Mechnization2/quaternion update ==
  data: omega_meas input; q_NB input; new_quat output; ST parameter
function new_quat = fcn(omega_meas, q_NB, ST)

% delta_angle = omega_meas .* ST;       % angle variation in 1 step
% delta_q = eul2quat([delta_angle(3), delta_angle(2), delta_angle(1)]);   % angle variation in quaternion form (rotation composition ZYX)
% 
% % Rotation composition as quaternion multiplication
% q_NB_p = q_multi(q_NB, delta_q);


omega_norm = norm(omega_meas);

if omega_norm < 1e-4  % or a small threshold
    delta_q = [1, 0, 0, 0];  % no rotation
else
    theta = double(omega_norm * ST);
    axis = double(omega_meas / omega_norm);
    delta_q = [cos(theta/2), axis' .* sin(theta/2)];
end

new_quat = quat_prod(q_NB,delta_q);
new_quat = new_quat / norm(new_quat);
end



function q = quat_prod(q1, q2)
    % q1, q2 are 1x4 vectors: [w x y z]
    w1 = q1(1); x1 = q1(2); y1 = q1(3); z1 = q1(4);
    w2 = q2(1); x2 = q2(2); y2 = q2(3); z2 = q2(4);

    w = w1*w2 - x1*x2 - y1*y2 - z1*z2;
    x = w1*x2 + x1*w2 + y1*z2 - z1*y2;
    y = w1*y2 - x1*z2 + y1*w2 + z1*x2;
    z = w1*z2 + x1*y2 - y1*x2 + z1*w2;

    q = [w, x, y, z];
end

== matlab function nav_filter/MATLAB Function2 ==
  data: acc_meas input; acc_body output; quat input; g parameter
function acc_body = fcn(acc_meas, quat,g)
q = quaternion(quat');
g_b = rotmat(q,"frame")*g;
acc_body = acc_meas+g_b;

== matlab function nav_filter/MATLAB Function3 ==
  data: quatk input; quatk output; quatk_1 input
function quatk = fcn(quatk, quatk_1)
if dot(quatk, quatk_1)<0
    quatk = -quatk;
end

== matlab function nav_filter/MATLAB Function1 ==
  data: quat_triad output; a_body_measured input; mag_body_measured input; quat_KF input; g parameter; sensor_covariances parameter; cov_TRIAD output
function [quat_triad, cov_TRIAD]    = estimate_attitude_triad(a_body_measured, mag_body_measured, quat_KF,g,sensor_covariances)
    
    % Reference vectors in NED (navigation frame)
    g_nav = [0; 0; 1];
    mag_nav = [0.4970; 0.0317; 0.8672];  % Adjust to local magnetic inclination if needed

    % Normalize sensor measurements
    mag_body = mag_body_measured / norm(mag_body_measured);


    if (norm(mag_body) < 1e-4)
        mag_body = [0.491 0.0323 0.8678]';
    end

    if 0.9*norm(g)<norm(a_body_measured) && norm(a_body_measured)<1.1*norm(g)
        g_body = -a_body_measured;

        if norm(g_body) < 1e-4
            g_body = [0; 0; 1]; % or some fallback gravity vector in body frame
        else
            g_body = g_body / norm(g_body);
        end

        % Construct TRIAD reference frame
        t1 = g_nav;
        t2 = cross(g_nav, mag_nav); t2 = t2 / norm(t2);
        t3 = cross(t1, t2);

        % Construct TRIAD body frame
        b1 = g_body;
        b2 = cross(g_body, mag_body); b2 = b2 / norm(b2);
        b3 = cross(b1, b2);
        
        % Convert rotation matrix to quaternion
        c = (b1*t1' + b2*t2' + b3*t3')';

        q1 = 0.5*sqrt(1+c(1,1)+c(2,2)+c(3,3));
        q2 = 0.25/q1*(c(3,2)-c(2,3));
        q3 = 0.25/q1*(c(1,3)-c(3,1));
        q4 = 0.25/q1*(c(2,1)-c(1,2));
        quat_triad = [q1 q2 q3 q4]';
        % q_out = [q1 q2 q3 q4]';
        % quat_triad = (double(rotm2quat(R)))'; % MATLAB gives [w x y z]
        quat_triad = quat_triad/norm(quat_triad);
        cov_TRIAD = sensor_covariances(10:13);


    else
        cov_TRIAD = sensor_covariances(10:13).*10;
        quat_triad = quat_KF;
    end


   
    if dot(quat_triad, quat_KF) < 0
        quat_triad = -quat_triad;
    end

    
end

== matlab function nav_filter/UWB sensor 10Hz/Distances computation ==
  data: pos input; d output; P_bases_ned parameter
function d = dist_comp(pos, P_bases_ned)
% Calcola le distanze tra la posizione stimata e ciascuna base UWB
%
% Input:
%   pos_ned:       vettore 3x1 [x; y; z]
%   P_bases_ned:   matrice Nx3 con le posizioni delle basi (ogni riga è una base)
%
% Output:
%   d:             vettore Nx1 con le distanze calcolate

N = size(P_bases_ned, 1);  % numero di basi
d = zeros(N, 1);

for i = 1:N
    Pi = P_bases_ned(i, :)';
    d(i) = norm(pos - Pi);
end

% function d = dist_comp(pos_ned, P_base1_ned, P_base2_ned, P_base3_ned, P_base4_ned)
% d = [ norm(pos_ned-P_base1_ned); 
%       norm(pos_ned-P_base2_ned);
%       norm(pos_ned-P_base3_ned);
%       norm(pos_ned-P_base4_ned) ];

== matlab function nav_filter/MATLAB Function ==
  data: Z output; d_UWB_measured input; acc_KF output; vel_KF output; pos_KF output; omega_KF output; quat_KF output; bias_gyro_KF output; Pout output; a_body_measured input; gyro_meas input; quat_triad input; ST parameter; g parameter; Q parameter; sensor_covariances parameter; P_bases_ned parameter; Flag50Hz input; pos parameter; vel_ned parameter; acc parameter; quat_nb parameter; pqr parameter; quat_KF_1 input; cov_TRIAD input
function [Z, acc_KF, vel_KF, pos_KF, omega_KF, quat_KF, bias_gyro_KF,Pout] = navigation_KF(d_UWB_measured, a_body_measured, gyro_meas, quat_triad, ...
                                                                                      ST, g, Q, sensor_covariances, P_bases_ned,Flag50Hz, pos,vel_ned,...
                                                                                      acc, quat_nb, pqr, quat_KF_1, cov_TRIAD)
% state vector - [pos(3), vel(3), acc(3), q(4), omega(3), gyro_bias(3)] -> 19-dim
% Measure = 13-dimensional vector
% measure = [UWB(pos_n, pos_e, pos_d), Acc (acc_x, acc_y, acc_z), Triad, gyro (wx, wy, wz)]

%% definition of variables
persistent P % covariance matrix 
persistent x 



if isempty(P)   % this is done in the first cycle --> the persistent variables are inititialized
    % P = single(0.1)*Q;
    % P(4:6,4:6) = P(4:6,4:6); % apriori esteem of velocity are bad
    % %P(9,9)=P(9,9)*1e5;
    % P(17:19,17:19) = P(17:19,17:19)*1e3; % apriori esteem of biases are bad
    % P(19,19) = P(19,19)*1e-2;
    P=Q;
    % P(10:13,10:13) = diag(1e-4);

    x = zeros(19,1);
    
    % x(1:3) = pos(1,:)';
    % x(7:9) = acc(1,:)';
    % x(4:6) = vel_ned(1,:)';
    % 
    % x(10:13) = quat_nb(1,:)';
    % x(14:16) = pqr(1,:)';
    % x(17:19) = ones(3,1);
    % x(4)=1.0536 ;
    % x(5)=0.1416;
    % x(6)=0.0002;
    % x(9)= -9.81;
    % 
    x(10) = 1; % element of the quaternion q_w = 1
    % x(13) = 0.7071;
    % 
   
  
end

%% Prediction
[x, P, F] = prediction(x, ST, Q, P, g);
 

%% Correction
measure = [d_UWB_measured; a_body_measured; quat_triad; gyro_meas];
[x, P, H] = correction(x, P, measure, sensor_covariances, g, P_bases_ned,Flag50Hz, quat_KF_1, cov_TRIAD);

% output
pos_KF = x(1:3);
vel_KF = x(4:6);
acc_KF = x(7:9);
quat_KF = x(10:13);
omega_KF = x(14:16);
bias_gyro_KF = x(17:19);

n = size(F, 1);  % number of states
O = [H];
for k = 1:n-1
    O = [O; H * F^k];
end
% if rank(O)<n
%     disp('perdita di rango');
%     disp(rank(O));
% end
Z = cond(O);
Pout = P;
end

% ----------------------------------------------------------------------------------

function [x, P, F] = prediction(x, dt, Q, P, g)
% update the predicted state
    north = x(1); east = x(2); down = x(3);         % pos (NED)
    vel_n = x(4); vel_e = x(5); vel_d = x(6);       % vel (nav frame)
    acc_x = x(7); acc_y = x(8); acc_z = x(9);       % acc (body frame)
    qw = x(10); qx = x(11); qy = x(12); qz = x(13); % quaternion (from nav to body)
    w_x = x(14); w_y = x(15); w_z = x(16);          % omega (body)
    byas_gx = x(17); byas_gy = x(18); byas_gz = x(19);% byass gyro

    % convert acc from body to navigation frame
    %R_nb = quat2rotm([qw, qx, qy, qz]);     % rotation from nav to body
    R_nb = [qw^2 + qx^2 - qy^2 - qz^2,     2*(qx*qy - qw*qz),           2*(qx*qz + qw*qy);
        2*(qx*qy + qw*qz),             qw^2 - qx^2 + qy^2 - qz^2,   2*(qy*qz - qw*qx);
        2*(qx*qz - qw*qy),             2*(qy*qz + qw*qx),           qw^2 - qx^2 - qy^2 + qz^2];

    acc_ned1 = R_nb' * [acc_x; acc_y; acc_z];
    
    acc_n = acc_ned1(1);
    acc_e = acc_ned1(2);
    acc_d = acc_ned1(3);
    
    
    % positions
    north = north + vel_n*dt + 0.5*acc_n*dt^2;
    east = east + vel_e*dt + 0.5*acc_e*dt^2 ;
    down = down + vel_d*dt + 0.5*acc_d*dt^2;

    % vel
    vel_n = vel_n + acc_n*dt;
    vel_e = vel_e + acc_e*dt;
    vel_d = vel_d + acc_d*dt;

    % attitude - quaternion update
    omega = [w_x, w_y, w_z];  % angular velocity
    omega_norm = norm(omega);

    if omega_norm < 1e-4  % or a small threshold
        delta_q = [1, 0, 0, 0];  % no rotation
    else
        theta = double(omega_norm * dt);
        axis = double(omega / omega_norm);
        delta_q = [cos(theta/2), axis .* sin(theta/2)];
    end
    
    new_quat = quat_prod([qw,qx,qy,qz],delta_q);
   
    new_quat = new_quat / norm(new_quat);
    % % if dot(new_quat, [qw,qx,qy,qz])<0
    % %     new_quat = -new_quat;
    % % end
    
    q_w = new_quat(1);
    q_x = new_quat(2);
    q_y = new_quat(3);
    q_z = new_quat(4);

    % output:
    x = [north, east, down, vel_n, vel_e, vel_d, acc_x, acc_y, acc_z, new_quat, w_x, w_y, w_z, byas_gx, byas_gy, byas_gz]';

    % P
    F = F_matrix(north,east,down,vel_n,vel_e,vel_d,acc_x,acc_y,acc_z,q_w,q_x,q_y,q_z,w_x,w_y,w_z,byas_gx,byas_gy,byas_gz,dt);
    P = F*P*F' + Q;
    
        
end
  
function [x, P, H] = correction(x, P, measure, covariances,g,P_bases_ned,Flag25Hz, quat_KF_1, cov_TRIAD)
    H_tot = H_matrix(x,P_bases_ned);
    y_pred_tot = get_y_pred(x,g,P_bases_ned);
    
    
    
    if Flag25Hz
        y = measure(1:end);
        y_pred = y_pred_tot(1:end);
        H = H_tot(1:end,:);
        R = diag(covariances);
        R(10:13,10:13) = diag(cov_TRIAD);
        
    else
        y = measure(end-9:end);
        y_pred = y_pred_tot(end-9:end);
        H = H_tot(end-9:end,:);
        R = diag(covariances(end-9:end));
        R(end-6:end-3,end-6:end-3)= diag(cov_TRIAD);
        
    end
    
    S = H*P*H' + R;
    % if dot(y_pred(end-6:end-3), y(end-6:end-3))<0
    %     y_pred(end-6:end-3) = -y_pred(end-6:end-3);
    % end
    e = y - y_pred;  
    disp(e(end-9:end-7));
    L = P*H'*pinv(S);
    corr = L*e;            
    x = x + corr;
    % % x(10:13) = x(10:13)/norm(x(10:13));
    P = (eye(19) - L*H)*P*(eye(19) - L*H)' + L*R*L';


    
   

end

function q = quat_prod(q1, q2)
    % q1, q2 are 1x4 vectors: [w x y z]
    w1 = q1(1); x1 = q1(2); y1 = q1(3); z1 = q1(4);
    w2 = q2(1); x2 = q2(2); y2 = q2(3); z2 = q2(4);

    w = w1*w2 - x1*x2 - y1*y2 - z1*z2;
    x = w1*x2 + x1*w2 + y1*z2 - z1*y2;
    y = w1*y2 - x1*z2 + y1*w2 + z1*x2;
    z = w1*z2 + x1*y2 - y1*x2 + z1*w2;

    q = [w, x, y, z];
end

== matlab function nav_filter/Magnetometer 50Hz/MATLAB Function2 ==
  data: u input; y output
function y = fcn(u)
disp(size(u));
y = u;
